simulink model "Modul_PV"  (R2023a)
settings: Solver=ode45  StartTime=0.0  StopTime=1  RelTol=1e-3
values from neighbouring files (symbols this model uses):
  Eg = 1.12    [paramsv1.m]
  Is = 2.16e-08    [paramsv1.m]
  Ki = 0.05    [PV_Params.mat]    (also in PVparamsforV3.m = 0.0005; paramsv1.m = 0.0017)
  N = 1.5    [paramsv1.m]
  Tn = 298.15    [paramsv1.m]
  Vt = 6.7084e+22    [paramsv1.m]
libraries: simulink x1
settings Model: Creator=lucea  LastModifiedBy=lucea

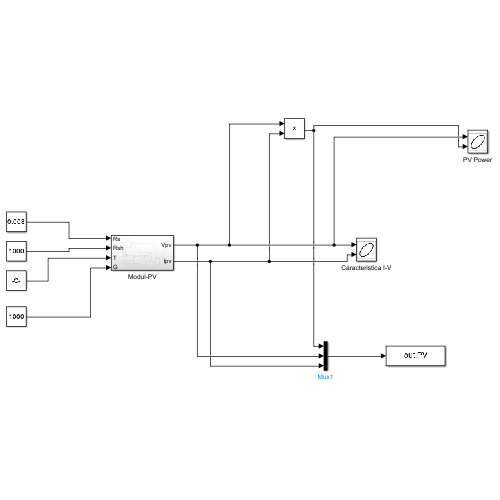
[thumbnail: Simulink's stored preview of the top-level diagram]
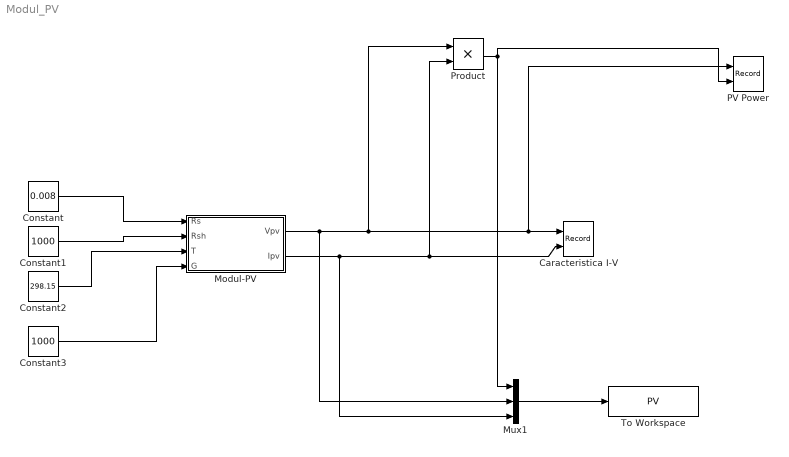
== system Modul_PV ==
  Caracteristica I-V : Record  FileSettingsInternal="{\"entries\":[{\"content\":{\"excelSettings\":{\"content\":{},\"type\":\"Streamout.ExcelSettings\"}},\"type\":\"Streamout.FileSettingStorage\",\"uuid\":\"\"}],\"packageUris\":[\"http:\\/\\/schema.mathworks.com\\/mf0\\/streamout_blocks\\/R2020a\"],\"version\":\"1.0\"}"  Layout=[1 1]  SignalsInternal="{\"entries\":[{\"content\":{\"signals\":[{\"content\":{\"blockPath\":[],\"dimensions\":[1],\"domain\":\"\",\"lineColor\":\"#edb120\",\"plots\":[1],\"port\":1,\"sid\":[\"\"],\"signalID\":768,\"signalName\":\"Modul-PV:1\"},\"type\":\"RecordBlkView.Signal\",\"uuid\":\"\"},{\"content\":{\"blockPath\":[],\"dimensions\":[1],\"domain\":\"\",\"lineColor\":\"#7e2f8e\",\"plots\":[1],\"port\":2,\"sid\":[\"\"],\"signalID\":772,\"signalName\":\"Modul-PV:2\"},\"type\":\"RecordBlkView.Signal\",\"uuid\":\"\"}]},\"type\":\"RecordBlkView.InputSignals\",\"uuid\":\"\"}],\"packageUris\":[\"http:\\/\\/schema.mathworks.com\\/mf0\\/streamout_blocks\\/R2020a\"],\"version\":\"1.0\"}"  VisualizationBindings="{\"xyplotplugin\":{\"info\":[{\"series\":[{\"bindingParametersList\":[{\"parameter\":\"X-Axis\",\"signalID\":768,\"signalName\":\"Modul-PV:1\"},{\"parameter\":\"Y-Axis\",\"signalID\":772,\"signalName\":\"Modul-PV:2\"}],\"seriesID\":7465}],\"subplotID\":1}]}}"  CompatibilityTag=XY  st=-1
  Constant : Constant  Value=0.008
  Constant1 : Constant  Value=1000
  Constant2 : Constant  Value=298.15
  Constant3 : Constant  Value=1000
  Modul-PV : Subsystem
  Mux1 : Mux  Inputs=3
  PV Power : Record  FileSettingsInternal="{\"entries\":[{\"content\":{\"excelSettings\":{\"content\":{},\"type\":\"Streamout.ExcelSettings\"}},\"type\":\"Streamout.FileSettingStorage\",\"uuid\":\"\"}],\"packageUris\":[\"http:\\/\\/schema.mathworks.com\\/mf0\\/streamout_blocks\\/R2020a\"],\"version\":\"1.0\"}"  Layout=[1 1]  SignalsInternal="{\"entries\":[{\"content\":{\"signals\":[{\"content\":{\"blockPath\":[],\"dimensions\":[1],\"domain\":\"\",\"lineColor\":\"#77ac30\",\"plots\":[1],\"port\":1,\"sid\":[\"\"],\"signalID\":776,\"signalName\":\"Modul-PV:1\"},\"type\":\"RecordBlkView.Signal\",\"uuid\":\"\"},{\"content\":{\"blockPath\":[],\"dimensions\":[1],\"domain\":\"\",\"lineColor\":\"#4dbeee\",\"plots\":[1],\"port\":2,\"sid\":[\"\"],\"signalID\":780,\"signalName\":\"Product\"},\"type\":\"RecordBlkView.Signal\",\"uuid\":\"\"}]},\"type\":\"RecordBlkView.InputSignals\",\"uuid\":\"\"}],\"packageUris\":[\"http:\\/\\/schema.mathworks.com\\/mf0\\/streamout_blocks\\/R2020a\"],\"version\":\"1.0\"}"  VisualizationBindings="{\"xyplotplugin\":{\"info\":[{\"series\":[{\"bindingParametersList\":[{\"parameter\":\"X-Axis\",\"signalID\":780,\"signalName\":\"Product\"},{\"parameter\":\"Y-Axis\",\"signalID\":776,\"signalName\":\"Modul-PV:1\"}],\"seriesID\":49836}],\"subplotID\":1}]}}"  CompatibilityTag=XY  st=-1
  Product : Product
  To Workspace : ToWorkspace  VariableName=PV  SaveFormat=Structure With Time  SampleTime=-1
  wires:
  Modul-PV/1(Vpv) -> Mux1/2, PV Power/1, Caracteristica I-V/1, Product/1
  Modul-PV/2(Ipv) -> Mux1/3, Caracteristica I-V/2, Product/2
  Product/1 -> PV Power/2, Mux1/1
  Mux1/1 -> To Workspace/1
  Constant/1 -> Modul-PV/1(Rs)
  Constant1/1 -> Modul-PV/2(Rsh)
  Constant2/1 -> Modul-PV/3(T)
  Constant3/1 -> Modul-PV/4(G)

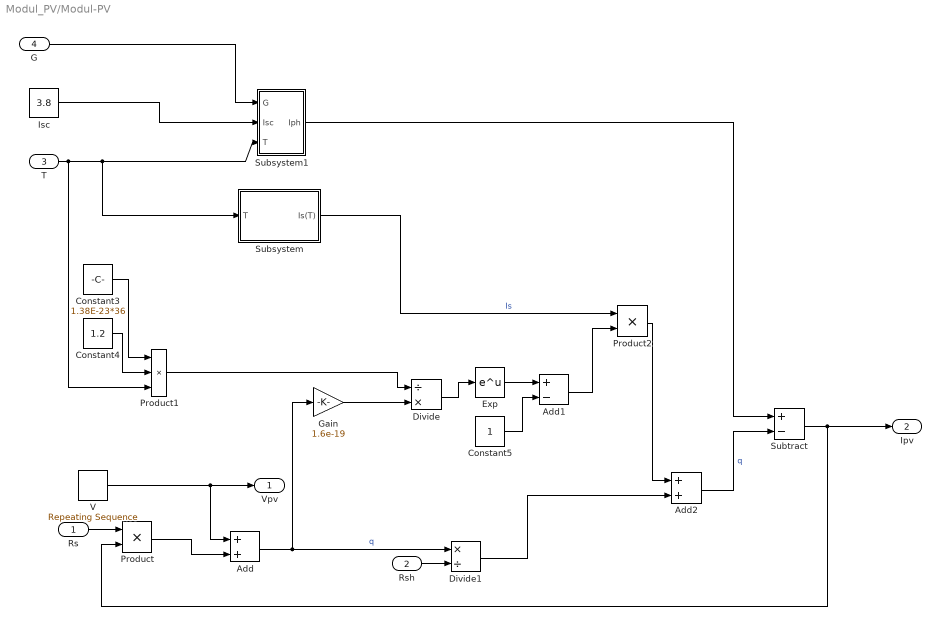
== system Modul_PV/Modul-PV ==
  Rs : Inport
  Rsh : Inport  Port=2
  T : Inport  Port=3
  G : Inport  Port=4
  Add : Sum
  Add1 : Sum  Inputs=+-
  Add2 : Sum
  Constant3 : Constant  Value=1.38E-23*36
  Constant4 : Constant  Value=1.2
  Constant5 : Constant
  Divide : Product  Inputs=/*
  Divide1 : Product  Inputs=*/
  Exp : Math
  Gain : Gain  Gain=1.6e-19
  Isc : Constant  Value=3.8
  Product : Product
  Product1 : Product  Inputs=3
  Product2 : Product
  Subsystem : Subsystem
  Subsystem1 : Subsystem
  Subtract : Sum  Inputs=+-
  V : simulink/Sources/Repeating Sequence  rep_seq_t=[0 1 2]  rep_seq_y=[-0.1 21.3 -0.1]
  Vpv : Outport
  Ipv : Outport  Port=2
  wires:
  T/1 -> Product1/3, Subsystem1/3(T), Subsystem/1(T)
  Divide/1 -> Exp/1
  Constant3/1 -> Product1/1
  Subtract/1 -> Ipv/1, Product/2
  Isc/1 -> Subsystem1/2(Isc)
  Add2/1 -> Subtract/2  "q"
  Constant4/1 -> Product1/2
  V/1 -> Vpv/1, Add/1
  Gain/1 -> Divide/2
  G/1 -> Subsystem1/1(G)
  Product/1 -> Add/2
  Add/1 -> Gain/1, Divide1/1  "q"
  Constant5/1 -> Add1/2
  Rs/1 -> Product/1
  Add1/1 -> Product2/2
  Subsystem/1(Is(T)) -> Product2/1  "Is"
  Exp/1 -> Add1/1
  Product2/1 -> Add2/1
  Rsh/1 -> Divide1/2
  Product1/1 -> Divide/1
  Divide1/1 -> Add2/2
  Subsystem1/1(Iph) -> Subtract/1

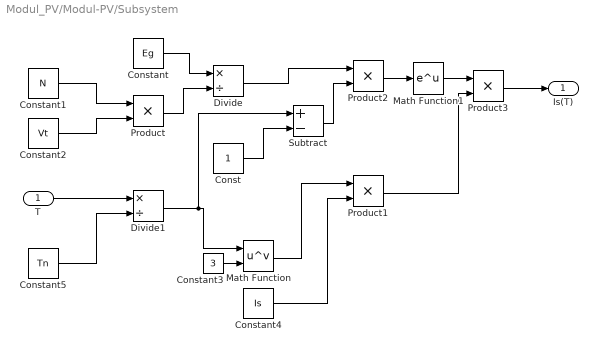
== system Modul_PV/Modul-PV/Subsystem ==
  T : Inport
  Const : Constant
  Constant : Constant  Value=Eg
  Constant1 : Constant  Value=N
  Constant2 : Constant  Value=Vt
  Constant3 : Constant  Value=3
  Constant4 : Constant  Value=Is
  Constant5 : Constant  Value=Tn
  Divide : Product  Inputs=*/
  Divide1 : Product  Inputs=*/
  Math Function : Math  Operator=pow  SignedPower=on
  Math Function1 : Math
  Product{,1..3} (4 alike) : Product
  Subtract : Sum  Inputs=+-
  Is(T) : Outport
  wires:
  Constant1/1 -> Product/1
  Divide/1 -> Product2/1
  Const/1 -> Subtract/2
  Divide1/1 -> Subtract/1, Math Function/1
  Constant4/1 -> Product1/2
  Constant2/1 -> Product/2
  Math Function1/1 -> Product3/1
  Product2/1 -> Math Function1/1
  Math Function/1 -> Product1/1
  Constant5/1 -> Divide1/2
  Subtract/1 -> Product2/2
  Product1/1 -> Product3/2
  T/1 -> Divide1/1
  Constant/1 -> Divide/1
  Product/1 -> Divide/2
  Constant3/1 -> Math Function/2
  Product3/1 -> Is(T)/1

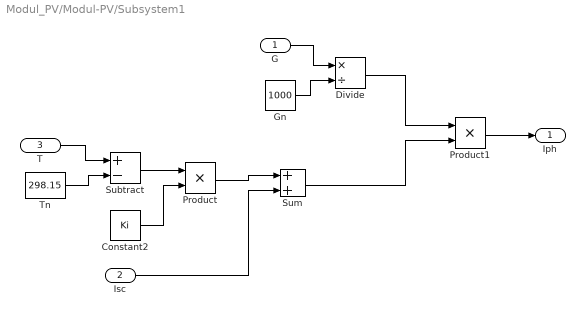
== system Modul_PV/Modul-PV/Subsystem1 ==
  G : Inport
  Isc : Inport  Port=2
  T : Inport  Port=3
  Constant2 : Constant  Value=Ki
  Divide : Product  Inputs=*/
  Gn : Constant  Value=1000
  Product : Product
  Product1 : Product
  Subtract : Sum  Inputs=+-
  Sum : Sum
  Tn : Constant  Value=298.15
  Iph : Outport
  wires:
  T/1 -> Subtract/1
  G/1 -> Divide/1
  Divide/1 -> Product1/1
  Product1/1 -> Iph/1
  Sum/1 -> Product1/2
  Product/1 -> Sum/1
  Tn/1 -> Subtract/2
  Constant2/1 -> Product/2
  Gn/1 -> Divide/2
  Isc/1 -> Sum/2
  Subtract/1 -> Product/1
